simulink model "station_no_recovery"  (R2015a)
settings: Solver=ode45  StartTime=0  StopTime=5000  FixedStep=10  MaxStep=1  RelTol=1e-3
(part 2 of 4)

== system station_no_recovery/Восстанавливаемые объекты/ГТЭ-6//6,3/Subsystem1 ==
  λ1 : Inport
  λ2 : Inport  Port=2
  M : Inport  Port=3
  dP : Inport  Port=4
  Pz : Inport  Port=5
  dt : Inport  Port=6
  trec : Inport  Port=7
  t_start : Inport  Port=8
  Chart : Stateflow chart  TreatAsAtomicUnit=on
  Clock : Clock
  Data Store Memory : DataStoreMemory  DataStoreName=t4_1
  Data Store Read : DataStoreRead  DataStoreName=t4_1
  Data Store Write : DataStoreWrite  DataStoreName=t4_1
  Display : Display
  Element Exponential : Subsystem  mask(Element Exponential){}
      mask help:
      | <p>Возвращает вероятность безотказной работы невосстанавливаемого элемента
      | по экспоненциальному закону распределения.</p>
      | <p>Экспоненциальное (или показательное) распределение — абсолютно непрерывное
      | распределение, моделирующее время между двумя последовательными свершениями
      | одного и того же события.</p>
      | <p>Экспоненциальное распределение используют при оценке надежности сложных
      | технических систем, не подверженных износу и старению и в случаях, когда
      | отказы объектов имеют случайный характер.</p>
      mask Help:
      | <p>Возвращает вероятность безотказной работы невосстанавливаемого элемента по экспоненциальному
      | закону распределения.</p>
      | <p>Экспоненциальное распределение используют при оценке надежности сложных
      | технических систем, не подверженных износу и старению и в случаях, когда
      | отказы объектов имеют случайный характер.</p>
      | <p>Входной параметр λ - интенсивность событий в рассматриваемом потоке.</p>
      | <p>Выходной параметр P(t) - вероятность безотказной работы элемента.</p>
      mask Display:
      | image('images/png/exp.png')
      | port_label('input', 1, 'λ')
      | port_label('output', 1, 'P(t)')
  Element Normal : Subsystem  mask(Element Normal){}
      mask help:
      | <p>Возвращает вероятность безотказной работы невосстанавливаемого
      | элемента по нормальному закону распределения.</p>
      | <p>Нормальное распределение, также называемое распределением Гаусса или
      | Гаусса — Лапласа — распределение вероятностей, которое в одномерном
      | случае задаётся функцией плотности вероятности, совпадающей с функцией
      | Гаусса.</p>
      | <p>Нормальное распределение обычно используют при оценке надежности объектов,
      | основной причиной отказа которых является износ.</p>
      mask Help:
      | <p>Возвращает вероятность безотказной работы невосстанавливаемого
      | элемента по нормальному закону распределения.</p>
      | <p>Нормальное распределение обычно используют при оценке надежности объектов,
      | основной причиной отказа которых является износ.</p>
      | <p>Входные параметры:</p>
      | <p>λ - среднее квадратическое отклонение наработки до отказа,</p>
      | <p>М - математическое ожидание наработки до отказа.</p>
      | <p>Выходной параметр P(t) - вероятность безотказной работы элемента.</p>
      mask Display:
      | image('images/png/normal_nogrid.png')
      | port_label('input', 1, 'λ')
      | port_label('input', 2, 'M')
      | port_label('output', 1, 'P(t)')
  Сircuit Series : Subsystem  mask(Сircuit Series){}
      mask help:
      | <p>Возвращает вероятность безотказной работы двух последовательно соединенных
      | элементов.</p>
      | <p>В системе с последовательной структурой отказ любого компонента приводит
      | к отказу системы в целом.</p>
      mask Help:
      | <p>Возвращает вероятность безотказной работы двух последовательно соединенных
      | элементов.</p>
      | <p>Входные параметры:</p>
      | <p>P1 - вероятность безотказной работы первого элемента,</p>
      | <p>P2 - вероятность безотказной работы второго элемента.</p>
      | <p>Выходной параметр P12 - вероятность безотказной работы двух последовательно
      | соединенных элементов.</p>
      mask Display:
      | image('images/png/series2.png')
      | port_label('input', 1, 'P1')
      | port_label('input', 2, 'P2')
      | port_label('output', 1, 'P12')
  P : Outport
  wires:
  M/1 -> Element Normal/2("M ")
  dP/1 -> Chart/5(dP)
  Pz/1 -> Chart/3(Pz)
  λ1/1 -> Element Exponential/1("lambda ")
  dt/1 -> Chart/2(delta_t)
  Clock/1 -> Chart/6(t)
  λ2/1 -> Element Normal/1("lambda ")
  Chart/2(P) -> P/1
  Element Normal/1(P(t)) -> Сircuit Series/2(P2)
  Element Exponential/1(P(t)1) -> Сircuit Series/1(P1)
  Сircuit Series/1(P12) -> Chart/7(P0), Display/1
  trec/1 -> Chart/4(trec)
  Chart/1(tv) -> Data Store Write/1
  t_start/1 -> Chart/1(t_start)
  Data Store Read/1 -> Element Exponential/2(t), Element Normal/3(t)

== system station_no_recovery/Восстанавливаемые объекты/ГТЭ-6//6,3/Subsystem2 ==
  λ1 : Inport
  λ2 : Inport  Port=2
  M : Inport  Port=3
  dP : Inport  Port=4
  Pz : Inport  Port=5
  dt : Inport  Port=6
  trec : Inport  Port=7
  t_start : Inport  Port=8
  Chart : Stateflow chart  TreatAsAtomicUnit=on
  Clock : Clock
  Data Store Memory : DataStoreMemory  DataStoreName=t4_2
  Data Store Read : DataStoreRead  DataStoreName=t4_2
  Data Store Write : DataStoreWrite  DataStoreName=t4_2
  Display : Display
  Element Exponential : Subsystem  mask(Element Exponential){}
      mask help:
      | <p>Возвращает вероятность безотказной работы невосстанавливаемого элемента
      | по экспоненциальному закону распределения.</p>
      | <p>Экспоненциальное (или показательное) распределение — абсолютно непрерывное
      | распределение, моделирующее время между двумя последовательными свершениями
      | одного и того же события.</p>
      | <p>Экспоненциальное распределение используют при оценке надежности сложных
      | технических систем, не подверженных износу и старению и в случаях, когда
      | отказы объектов имеют случайный характер.</p>
      mask Help:
      | <p>Возвращает вероятность безотказной работы невосстанавливаемого элемента по экспоненциальному
      | закону распределения.</p>
      | <p>Экспоненциальное распределение используют при оценке надежности сложных
      | технических систем, не подверженных износу и старению и в случаях, когда
      | отказы объектов имеют случайный характер.</p>
      | <p>Входной параметр λ - интенсивность событий в рассматриваемом потоке.</p>
      | <p>Выходной параметр P(t) - вероятность безотказной работы элемента.</p>
      mask Display:
      | image('images/png/exp.png')
      | port_label('input', 1, 'λ')
      | port_label('output', 1, 'P(t)')
  Element Normal : Subsystem  mask(Element Normal){}
      mask help:
      | <p>Возвращает вероятность безотказной работы невосстанавливаемого
      | элемента по нормальному закону распределения.</p>
      | <p>Нормальное распределение, также называемое распределением Гаусса или
      | Гаусса — Лапласа — распределение вероятностей, которое в одномерном
      | случае задаётся функцией плотности вероятности, совпадающей с функцией
      | Гаусса.</p>
      | <p>Нормальное распределение обычно используют при оценке надежности объектов,
      | основной причиной отказа которых является износ.</p>
      mask Help:
      | <p>Возвращает вероятность безотказной работы невосстанавливаемого
      | элемента по нормальному закону распределения.</p>
      | <p>Нормальное распределение обычно используют при оценке надежности объектов,
      | основной причиной отказа которых является износ.</p>
      | <p>Входные параметры:</p>
      | <p>λ - среднее квадратическое отклонение наработки до отказа,</p>
      | <p>М - математическое ожидание наработки до отказа.</p>
      | <p>Выходной параметр P(t) - вероятность безотказной работы элемента.</p>
      mask Display:
      | image('images/png/normal_nogrid.png')
      | port_label('input', 1, 'λ')
      | port_label('input', 2, 'M')
      | port_label('output', 1, 'P(t)')
  Сircuit Series : Subsystem  mask(Сircuit Series){}
      mask help:
      | <p>Возвращает вероятность безотказной работы двух последовательно соединенных
      | элементов.</p>
      | <p>В системе с последовательной структурой отказ любого компонента приводит
      | к отказу системы в целом.</p>
      mask Help:
      | <p>Возвращает вероятность безотказной работы двух последовательно соединенных
      | элементов.</p>
      | <p>Входные параметры:</p>
      | <p>P1 - вероятность безотказной работы первого элемента,</p>
      | <p>P2 - вероятность безотказной работы второго элемента.</p>
      | <p>Выходной параметр P12 - вероятность безотказной работы двух последовательно
      | соединенных элементов.</p>
      mask Display:
      | image('images/png/series2.png')
      | port_label('input', 1, 'P1')
      | port_label('input', 2, 'P2')
      | port_label('output', 1, 'P12')
  P : Outport
  wires:
  Data Store Read/1 -> Element Normal/3(t), Element Exponential/2(t)
  t_start/1 -> Chart/1(t_start)
  Chart/1(tv) -> Data Store Write/1
  trec/1 -> Chart/4(trec)
  Сircuit Series/1(P12) -> Display/1, Chart/7(P0)
  Element Exponential/1(P(t)1) -> Сircuit Series/1(P1)
  Element Normal/1(P(t)) -> Сircuit Series/2(P2)
  Chart/2(P) -> P/1
  λ2/1 -> Element Normal/1("lambda ")
  Clock/1 -> Chart/6(t)
  dt/1 -> Chart/2(delta_t)
  λ1/1 -> Element Exponential/1("lambda ")
  Pz/1 -> Chart/3(Pz)
  dP/1 -> Chart/5(dP)
  M/1 -> Element Normal/2("M ")

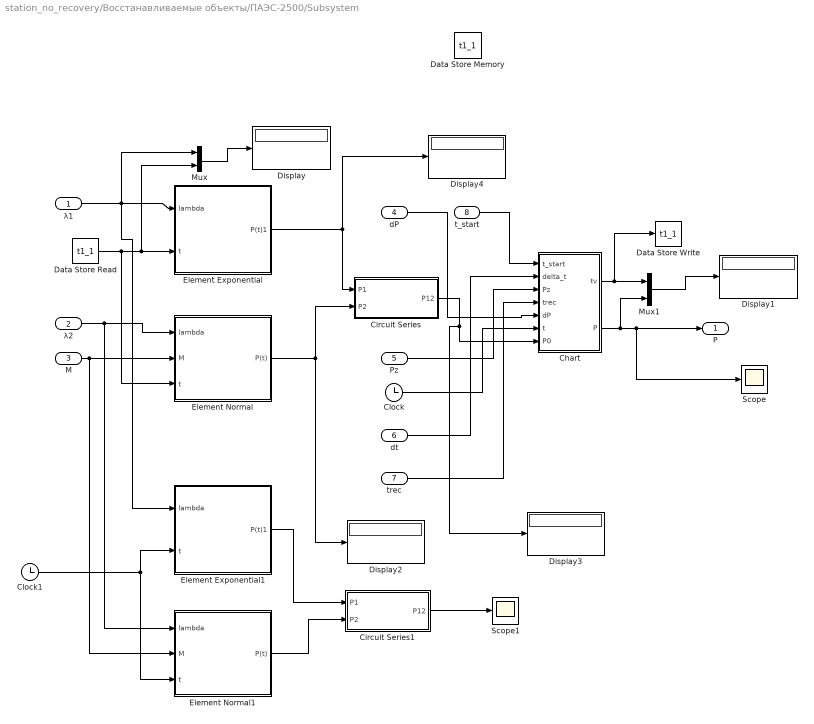
== system station_no_recovery/Восстанавливаемые объекты/ПАЭС-2500/Subsystem ==
  λ1 : Inport
  λ2 : Inport  Port=2
  M : Inport  Port=3
  dP : Inport  Port=4
  Pz : Inport  Port=5
  dt : Inport  Port=6
  trec : Inport  Port=7
  t_start : Inport  Port=8
  Chart : Stateflow chart  TreatAsAtomicUnit=on
  Clock : Clock
  Clock1 : Clock
  Data Store Memory : DataStoreMemory  DataStoreName=t1_1
  Data Store Read : DataStoreRead  DataStoreName=t1_1
  Data Store Write : DataStoreWrite  DataStoreName=t1_1
  Display{,1..4} (5 alike) : Display
  Element Exponential : Subsystem  mask(Element Exponential){}
      mask help:
      | <p>Возвращает вероятность безотказной работы невосстанавливаемого элемента
      | по экспоненциальному закону распределения.</p>
      | <p>Экспоненциальное (или показательное) распределение — абсолютно непрерывное
      | распределение, моделирующее время между двумя последовательными свершениями
      | одного и того же события.</p>
      | <p>Экспоненциальное распределение используют при оценке надежности сложных
      | технических систем, не подверженных износу и старению и в случаях, когда
      | отказы объектов имеют случайный характер.</p>
      mask Help:
      | <p>Возвращает вероятность безотказной работы невосстанавливаемого элемента по экспоненциальному
      | закону распределения.</p>
      | <p>Экспоненциальное распределение используют при оценке надежности сложных
      | технических систем, не подверженных износу и старению и в случаях, когда
      | отказы объектов имеют случайный характер.</p>
      | <p>Входной параметр λ - интенсивность событий в рассматриваемом потоке.</p>
      | <p>Выходной параметр P(t) - вероятность безотказной работы элемента.</p>
      mask Display:
      | image('images/png/exp.png')
      | port_label('input', 1, 'λ')
      | port_label('output', 1, 'P(t)')
  Element Exponential1 : Subsystem  mask(Element Exponential){}
      mask help:
      | <p>Возвращает вероятность безотказной работы невосстанавливаемого элемента
      | по экспоненциальному закону распределения.</p>
      | <p>Экспоненциальное (или показательное) распределение — абсолютно непрерывное
      | распределение, моделирующее время между двумя последовательными свершениями
      | одного и того же события.</p>
      | <p>Экспоненциальное распределение используют при оценке надежности сложных
      | технических систем, не подверженных износу и старению и в случаях, когда
      | отказы объектов имеют случайный характер.</p>
      mask Help:
      | <p>Возвращает вероятность безотказной работы невосстанавливаемого элемента по экспоненциальному
      | закону распределения.</p>
      | <p>Экспоненциальное распределение используют при оценке надежности сложных
      | технических систем, не подверженных износу и старению и в случаях, когда
      | отказы объектов имеют случайный характер.</p>
      | <p>Входной параметр λ - интенсивность событий в рассматриваемом потоке.</p>
      | <p>Выходной параметр P(t) - вероятность безотказной работы элемента.</p>
      mask Display:
      | image('images/png/exp.png')
      | port_label('input', 1, 'λ')
      | port_label('output', 1, 'P(t)')
  Element Normal : Subsystem  mask(Element Normal){}
      mask help:
      | <p>Возвращает вероятность безотказной работы невосстанавливаемого
      | элемента по нормальному закону распределения.</p>
      | <p>Нормальное распределение, также называемое распределением Гаусса или
      | Гаусса — Лапласа — распределение вероятностей, которое в одномерном
      | случае задаётся функцией плотности вероятности, совпадающей с функцией
      | Гаусса.</p>
      | <p>Нормальное распределение обычно используют при оценке надежности объектов,
      | основной причиной отказа которых является износ.</p>
      mask Help:
      | <p>Возвращает вероятность безотказной работы невосстанавливаемого
      | элемента по нормальному закону распределения.</p>
      | <p>Нормальное распределение обычно используют при оценке надежности объектов,
      | основной причиной отказа которых является износ.</p>
      | <p>Входные параметры:</p>
      | <p>λ - среднее квадратическое отклонение наработки до отказа,</p>
      | <p>М - математическое ожидание наработки до отказа.</p>
      | <p>Выходной параметр P(t) - вероятность безотказной работы элемента.</p>
      mask Display:
      | image('images/png/normal_nogrid.png')
      | port_label('input', 1, 'λ')
      | port_label('input', 2, 'M')
      | port_label('output', 1, 'P(t)')
  Element Normal1 : Subsystem  mask(Element Normal){}
      mask help:
      | <p>Возвращает вероятность безотказной работы невосстанавливаемого
      | элемента по нормальному закону распределения.</p>
      | <p>Нормальное распределение, также называемое распределением Гаусса или
      | Гаусса — Лапласа — распределение вероятностей, которое в одномерном
      | случае задаётся функцией плотности вероятности, совпадающей с функцией
      | Гаусса.</p>
      | <p>Нормальное распределение обычно используют при оценке надежности объектов,
      | основной причиной отказа которых является износ.</p>
      mask Help:
      | <p>Возвращает вероятность безотказной работы невосстанавливаемого
      | элемента по нормальному закону распределения.</p>
      | <p>Нормальное распределение обычно используют при оценке надежности объектов,
      | основной причиной отказа которых является износ.</p>
      | <p>Входные параметры:</p>
      | <p>λ - среднее квадратическое отклонение наработки до отказа,</p>
      | <p>М - математическое ожидание наработки до отказа.</p>
      | <p>Выходной параметр P(t) - вероятность безотказной работы элемента.</p>
      mask Display:
      | image('images/png/normal_nogrid.png')
      | port_label('input', 1, 'λ')
      | port_label('input', 2, 'M')
      | port_label('output', 1, 'P(t)')
  Mux : Mux  Inputs=2
  Mux1 : Mux  Inputs=2
  Scope : Scope
  Scope1 : Scope
      settings: SaveName=ScopeData2
  Сircuit Series : Subsystem  mask(Сircuit Series){}
      mask help:
      | <p>Возвращает вероятность безотказной работы двух последовательно соединенных
      | элементов.</p>
      | <p>В системе с последовательной структурой отказ любого компонента приводит
      | к отказу системы в целом.</p>
      mask Help:
      | <p>Возвращает вероятность безотказной работы двух последовательно соединенных
      | элементов.</p>
      | <p>Входные параметры:</p>
      | <p>P1 - вероятность безотказной работы первого элемента,</p>
      | <p>P2 - вероятность безотказной работы второго элемента.</p>
      | <p>Выходной параметр P12 - вероятность безотказной работы двух последовательно
      | соединенных элементов.</p>
      mask Display:
      | image('images/png/series2.png')
      | port_label('input', 1, 'P1')
      | port_label('input', 2, 'P2')
      | port_label('output', 1, 'P12')
  Сircuit Series1 : Subsystem  mask(Сircuit Series){}
      mask help:
      | <p>Возвращает вероятность безотказной работы двух последовательно соединенных
      | элементов.</p>
      | <p>В системе с последовательной структурой отказ любого компонента приводит
      | к отказу системы в целом.</p>
      mask Help:
      | <p>Возвращает вероятность безотказной работы двух последовательно соединенных
      | элементов.</p>
      | <p>Входные параметры:</p>
      | <p>P1 - вероятность безотказной работы первого элемента,</p>
      | <p>P2 - вероятность безотказной работы второго элемента.</p>
      | <p>Выходной параметр P12 - вероятность безотказной работы двух последовательно
      | соединенных элементов.</p>
      mask Display:
      | image('images/png/series2.png')
      | port_label('input', 1, 'P1')
      | port_label('input', 2, 'P2')
      | port_label('output', 1, 'P12')
  P : Outport
  wires:
  Element Exponential/1(P(t)1) -> Сircuit Series/1(P1), Display4/1
  Element Normal/1(P(t)) -> Сircuit Series/2(P2), Display2/1
  Chart/1(tv) -> Data Store Write/1, Mux1/1
  Chart/2(P) -> Mux1/2, Scope/1, P/1
  λ2/1 -> Element Normal1/1("lambda "), Element Normal/1("lambda ")
  Сircuit Series/1(P12) -> Chart/7(P0), Display3/1
  λ1/1 -> Element Exponential1/1("lambda "), Mux/1, Element Exponential/1("lambda ")
  M/1 -> Element Normal1/2("M "), Element Normal/2("M ")
  Mux/1 -> Display/1
  Mux1/1 -> Display1/1
  t_start/1 -> Chart/1(t_start)
  dt/1 -> Chart/2(delta_t)
  Pz/1 -> Chart/3(Pz)
  trec/1 -> Chart/4(trec)
  Clock/1 -> Chart/6(t)
  dP/1 -> Chart/5(dP)
  Data Store Read/1 -> Element Normal/3(t), Mux/2, Element Exponential/2(t)
  Clock1/1 -> Element Normal1/3(t), Element Exponential1/2(t)
  Element Exponential1/1(P(t)1) -> Сircuit Series1/1(P1)
  Element Normal1/1(P(t)) -> Сircuit Series1/2(P2)
  Сircuit Series1/1(P12) -> Scope1/1

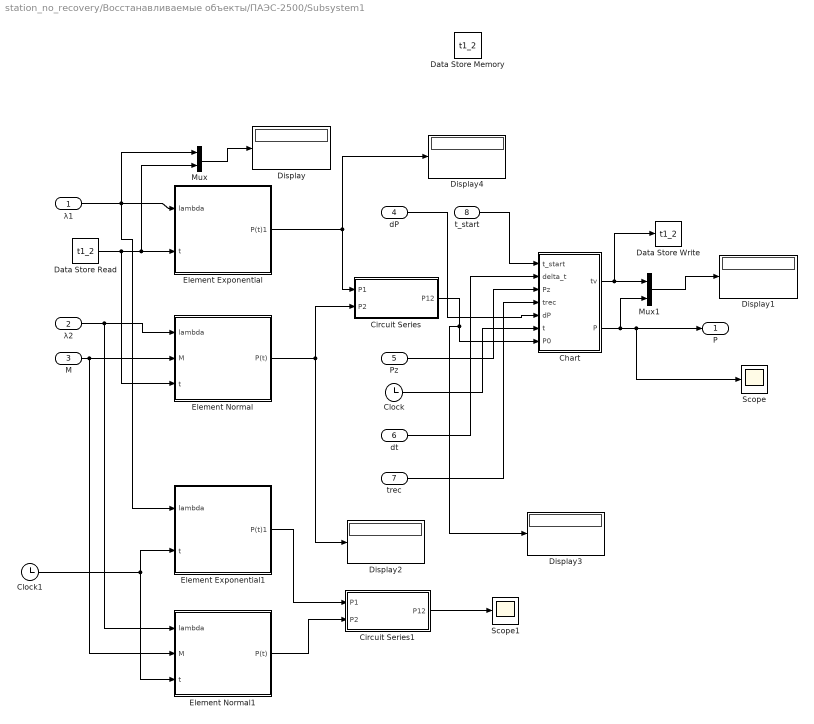
== system station_no_recovery/Восстанавливаемые объекты/ПАЭС-2500/Subsystem1 ==
  λ1 : Inport
  λ2 : Inport  Port=2
  M : Inport  Port=3
  dP : Inport  Port=4
  Pz : Inport  Port=5
  dt : Inport  Port=6
  trec : Inport  Port=7
  t_start : Inport  Port=8
  Chart : Stateflow chart  TreatAsAtomicUnit=on
  Clock : Clock
  Clock1 : Clock
  Data Store Memory : DataStoreMemory  DataStoreName=t1_2
  Data Store Read : DataStoreRead  DataStoreName=t1_2
  Data Store Write : DataStoreWrite  DataStoreName=t1_2
  Display{,1..4} (5 alike) : Display
  Element Exponential : Subsystem  mask(Element Exponential){}
      mask help:
      | <p>Возвращает вероятность безотказной работы невосстанавливаемого элемента
      | по экспоненциальному закону распределения.</p>
      | <p>Экспоненциальное (или показательное) распределение — абсолютно непрерывное
      | распределение, моделирующее время между двумя последовательными свершениями
      | одного и того же события.</p>
      | <p>Экспоненциальное распределение используют при оценке надежности сложных
      | технических систем, не подверженных износу и старению и в случаях, когда
      | отказы объектов имеют случайный характер.</p>
      mask Help:
      | <p>Возвращает вероятность безотказной работы невосстанавливаемого элемента по экспоненциальному
      | закону распределения.</p>
      | <p>Экспоненциальное распределение используют при оценке надежности сложных
      | технических систем, не подверженных износу и старению и в случаях, когда
      | отказы объектов имеют случайный характер.</p>
      | <p>Входной параметр λ - интенсивность событий в рассматриваемом потоке.</p>
      | <p>Выходной параметр P(t) - вероятность безотказной работы элемента.</p>
      mask Display:
      | image('images/png/exp.png')
      | port_label('input', 1, 'λ')
      | port_label('output', 1, 'P(t)')
  Element Exponential1 : Subsystem  mask(Element Exponential){}
      mask help:
      | <p>Возвращает вероятность безотказной работы невосстанавливаемого элемента
      | по экспоненциальному закону распределения.</p>
      | <p>Экспоненциальное (или показательное) распределение — абсолютно непрерывное
      | распределение, моделирующее время между двумя последовательными свершениями
      | одного и того же события.</p>
      | <p>Экспоненциальное распределение используют при оценке надежности сложных
      | технических систем, не подверженных износу и старению и в случаях, когда
      | отказы объектов имеют случайный характер.</p>
      mask Help:
      | <p>Возвращает вероятность безотказной работы невосстанавливаемого элемента по экспоненциальному
      | закону распределения.</p>
      | <p>Экспоненциальное распределение используют при оценке надежности сложных
      | технических систем, не подверженных износу и старению и в случаях, когда
      | отказы объектов имеют случайный характер.</p>
      | <p>Входной параметр λ - интенсивность событий в рассматриваемом потоке.</p>
      | <p>Выходной параметр P(t) - вероятность безотказной работы элемента.</p>
      mask Display:
      | image('images/png/exp.png')
      | port_label('input', 1, 'λ')
      | port_label('output', 1, 'P(t)')
  Element Normal : Subsystem  mask(Element Normal){}
      mask help:
      | <p>Возвращает вероятность безотказной работы невосстанавливаемого
      | элемента по нормальному закону распределения.</p>
      | <p>Нормальное распределение, также называемое распределением Гаусса или
      | Гаусса — Лапласа — распределение вероятностей, которое в одномерном
      | случае задаётся функцией плотности вероятности, совпадающей с функцией
      | Гаусса.</p>
      | <p>Нормальное распределение обычно используют при оценке надежности объектов,
      | основной причиной отказа которых является износ.</p>
      mask Help:
      | <p>Возвращает вероятность безотказной работы невосстанавливаемого
      | элемента по нормальному закону распределения.</p>
      | <p>Нормальное распределение обычно используют при оценке надежности объектов,
      | основной причиной отказа которых является износ.</p>
      | <p>Входные параметры:</p>
      | <p>λ - среднее квадратическое отклонение наработки до отказа,</p>
      | <p>М - математическое ожидание наработки до отказа.</p>
      | <p>Выходной параметр P(t) - вероятность безотказной работы элемента.</p>
      mask Display:
      | image('images/png/normal_nogrid.png')
      | port_label('input', 1, 'λ')
      | port_label('input', 2, 'M')
      | port_label('output', 1, 'P(t)')
  Element Normal1 : Subsystem  mask(Element Normal){}
      mask help:
      | <p>Возвращает вероятность безотказной работы невосстанавливаемого
      | элемента по нормальному закону распределения.</p>
      | <p>Нормальное распределение, также называемое распределением Гаусса или
      | Гаусса — Лапласа — распределение вероятностей, которое в одномерном
      | случае задаётся функцией плотности вероятности, совпадающей с функцией
      | Гаусса.</p>
      | <p>Нормальное распределение обычно используют при оценке надежности объектов,
      | основной причиной отказа которых является износ.</p>
      mask Help:
      | <p>Возвращает вероятность безотказной работы невосстанавливаемого
      | элемента по нормальному закону распределения.</p>
      | <p>Нормальное распределение обычно используют при оценке надежности объектов,
      | основной причиной отказа которых является износ.</p>
      | <p>Входные параметры:</p>
      | <p>λ - среднее квадратическое отклонение наработки до отказа,</p>
      | <p>М - математическое ожидание наработки до отказа.</p>
      | <p>Выходной параметр P(t) - вероятность безотказной работы элемента.</p>
      mask Display:
      | image('images/png/normal_nogrid.png')
      | port_label('input', 1, 'λ')
      | port_label('input', 2, 'M')
      | port_label('output', 1, 'P(t)')
  Mux : Mux  Inputs=2
  Mux1 : Mux  Inputs=2
  Scope : Scope
  Scope1 : Scope
      settings: SaveName=ScopeData2
  Сircuit Series : Subsystem  mask(Сircuit Series){}
      mask help:
      | <p>Возвращает вероятность безотказной работы двух последовательно соединенных
      | элементов.</p>
      | <p>В системе с последовательной структурой отказ любого компонента приводит
      | к отказу системы в целом.</p>
      mask Help:
      | <p>Возвращает вероятность безотказной работы двух последовательно соединенных
      | элементов.</p>
      | <p>Входные параметры:</p>
      | <p>P1 - вероятность безотказной работы первого элемента,</p>
      | <p>P2 - вероятность безотказной работы второго элемента.</p>
      | <p>Выходной параметр P12 - вероятность безотказной работы двух последовательно
      | соединенных элементов.</p>
      mask Display:
      | image('images/png/series2.png')
      | port_label('input', 1, 'P1')
      | port_label('input', 2, 'P2')
      | port_label('output', 1, 'P12')
  Сircuit Series1 : Subsystem  mask(Сircuit Series){}
      mask help:
      | <p>Возвращает вероятность безотказной работы двух последовательно соединенных
      | элементов.</p>
      | <p>В системе с последовательной структурой отказ любого компонента приводит
      | к отказу системы в целом.</p>
      mask Help:
      | <p>Возвращает вероятность безотказной работы двух последовательно соединенных
      | элементов.</p>
      | <p>Входные параметры:</p>
      | <p>P1 - вероятность безотказной работы первого элемента,</p>
      | <p>P2 - вероятность безотказной работы второго элемента.</p>
      | <p>Выходной параметр P12 - вероятность безотказной работы двух последовательно
      | соединенных элементов.</p>
      mask Display:
      | image('images/png/series2.png')
      | port_label('input', 1, 'P1')
      | port_label('input', 2, 'P2')
      | port_label('output', 1, 'P12')
  P : Outport
  wires:
  Сircuit Series1/1(P12) -> Scope1/1
  Element Normal1/1(P(t)) -> Сircuit Series1/2(P2)
  Element Exponential1/1(P(t)1) -> Сircuit Series1/1(P1)
  Clock1/1 -> Element Exponential1/2(t), Element Normal1/3(t)
  Data Store Read/1 -> Element Exponential/2(t), Mux/2, Element Normal/3(t)
  dP/1 -> Chart/5(dP)
  Clock/1 -> Chart/6(t)
  trec/1 -> Chart/4(trec)
  Pz/1 -> Chart/3(Pz)
  dt/1 -> Chart/2(delta_t)
  t_start/1 -> Chart/1(t_start)
  Mux1/1 -> Display1/1
  Mux/1 -> Display/1
  M/1 -> Element Normal/2("M "), Element Normal1/2("M ")
  λ1/1 -> Element Exponential/1("lambda "), Mux/1, Element Exponential1/1("lambda ")
  Сircuit Series/1(P12) -> Display3/1, Chart/7(P0)
  λ2/1 -> Element Normal/1("lambda "), Element Normal1/1("lambda ")
  Chart/2(P) -> P/1, Scope/1, Mux1/2
  Chart/1(tv) -> Mux1/1, Data Store Write/1
  Element Normal/1(P(t)) -> Display2/1, Сircuit Series/2(P2)
  Element Exponential/1(P(t)1) -> Display4/1, Сircuit Series/1(P1)

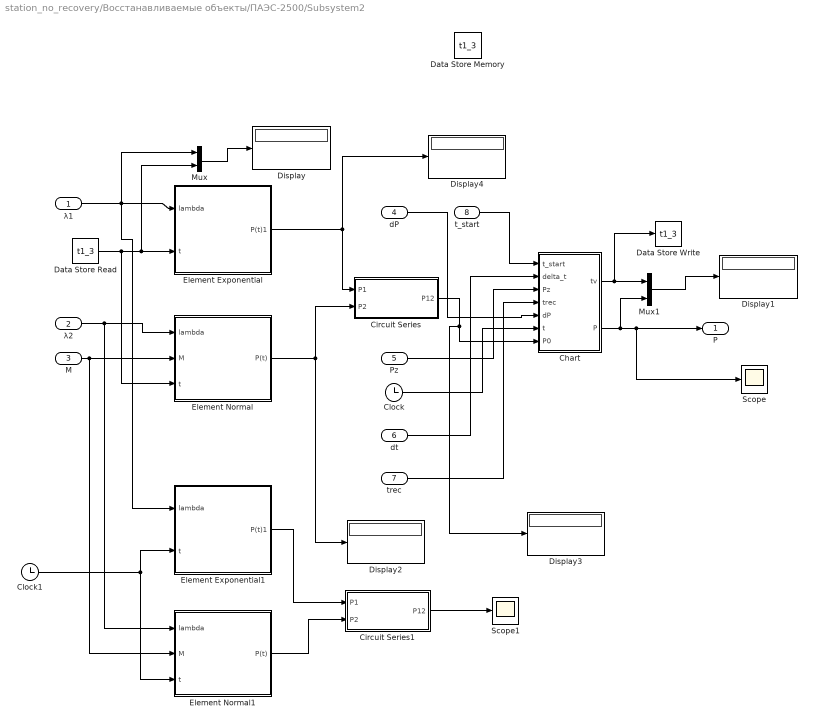
== system station_no_recovery/Восстанавливаемые объекты/ПАЭС-2500/Subsystem2 ==
  λ1 : Inport
  λ2 : Inport  Port=2
  M : Inport  Port=3
  dP : Inport  Port=4
  Pz : Inport  Port=5
  dt : Inport  Port=6
  trec : Inport  Port=7
  t_start : Inport  Port=8
  Chart : Stateflow chart  TreatAsAtomicUnit=on
  Clock : Clock
  Clock1 : Clock
  Data Store Memory : DataStoreMemory  DataStoreName=t1_3
  Data Store Read : DataStoreRead  DataStoreName=t1_3
  Data Store Write : DataStoreWrite  DataStoreName=t1_3
  Display{,1..4} (5 alike) : Display
  Element Exponential : Subsystem  mask(Element Exponential){}
      mask help:
      | <p>Возвращает вероятность безотказной работы невосстанавливаемого элемента
      | по экспоненциальному закону распределения.</p>
      | <p>Экспоненциальное (или показательное) распределение — абсолютно непрерывное
      | распределение, моделирующее время между двумя последовательными свершениями
      | одного и того же события.</p>
      | <p>Экспоненциальное распределение используют при оценке надежности сложных
      | технических систем, не подверженных износу и старению и в случаях, когда
      | отказы объектов имеют случайный характер.</p>
      mask Help:
      | <p>Возвращает вероятность безотказной работы невосстанавливаемого элемента по экспоненциальному
      | закону распределения.</p>
      | <p>Экспоненциальное распределение используют при оценке надежности сложных
      | технических систем, не подверженных износу и старению и в случаях, когда
      | отказы объектов имеют случайный характер.</p>
      | <p>Входной параметр λ - интенсивность событий в рассматриваемом потоке.</p>
      | <p>Выходной параметр P(t) - вероятность безотказной работы элемента.</p>
      mask Display:
      | image('images/png/exp.png')
      | port_label('input', 1, 'λ')
      | port_label('output', 1, 'P(t)')
  Element Exponential1 : Subsystem  mask(Element Exponential){}
      mask help:
      | <p>Возвращает вероятность безотказной работы невосстанавливаемого элемента
      | по экспоненциальному закону распределения.</p>
      | <p>Экспоненциальное (или показательное) распределение — абсолютно непрерывное
      | распределение, моделирующее время между двумя последовательными свершениями
      | одного и того же события.</p>
      | <p>Экспоненциальное распределение используют при оценке надежности сложных
      | технических систем, не подверженных износу и старению и в случаях, когда
      | отказы объектов имеют случайный характер.</p>
      mask Help:
      | <p>Возвращает вероятность безотказной работы невосстанавливаемого элемента по экспоненциальному
      | закону распределения.</p>
      | <p>Экспоненциальное распределение используют при оценке надежности сложных
      | технических систем, не подверженных износу и старению и в случаях, когда
      | отказы объектов имеют случайный характер.</p>
      | <p>Входной параметр λ - интенсивность событий в рассматриваемом потоке.</p>
      | <p>Выходной параметр P(t) - вероятность безотказной работы элемента.</p>
      mask Display:
      | image('images/png/exp.png')
      | port_label('input', 1, 'λ')
      | port_label('output', 1, 'P(t)')
  Element Normal : Subsystem  mask(Element Normal){}
      mask help:
      | <p>Возвращает вероятность безотказной работы невосстанавливаемого
      | элемента по нормальному закону распределения.</p>
      | <p>Нормальное распределение, также называемое распределением Гаусса или
      | Гаусса — Лапласа — распределение вероятностей, которое в одномерном
      | случае задаётся функцией плотности вероятности, совпадающей с функцией
      | Гаусса.</p>
      | <p>Нормальное распределение обычно используют при оценке надежности объектов,
      | основной причиной отказа которых является износ.</p>
      mask Help:
      | <p>Возвращает вероятность безотказной работы невосстанавливаемого
      | элемента по нормальному закону распределения.</p>
      | <p>Нормальное распределение обычно используют при оценке надежности объектов,
      | основной причиной отказа которых является износ.</p>
      | <p>Входные параметры:</p>
      | <p>λ - среднее квадратическое отклонение наработки до отказа,</p>
      | <p>М - математическое ожидание наработки до отказа.</p>
      | <p>Выходной параметр P(t) - вероятность безотказной работы элемента.</p>
      mask Display:
      | image('images/png/normal_nogrid.png')
      | port_label('input', 1, 'λ')
      | port_label('input', 2, 'M')
      | port_label('output', 1, 'P(t)')
  Element Normal1 : Subsystem  mask(Element Normal){}
      mask help:
      | <p>Возвращает вероятность безотказной работы невосстанавливаемого
      | элемента по нормальному закону распределения.</p>
      | <p>Нормальное распределение, также называемое распределением Гаусса или
      | Гаусса — Лапласа — распределение вероятностей, которое в одномерном
      | случае задаётся функцией плотности вероятности, совпадающей с функцией
      | Гаусса.</p>
      | <p>Нормальное распределение обычно используют при оценке надежности объектов,
      | основной причиной отказа которых является износ.</p>
      mask Help:
      | <p>Возвращает вероятность безотказной работы невосстанавливаемого
      | элемента по нормальному закону распределения.</p>
      | <p>Нормальное распределение обычно используют при оценке надежности объектов,
      | основной причиной отказа которых является износ.</p>
      | <p>Входные параметры:</p>
      | <p>λ - среднее квадратическое отклонение наработки до отказа,</p>
      | <p>М - математическое ожидание наработки до отказа.</p>
      | <p>Выходной параметр P(t) - вероятность безотказной работы элемента.</p>
      mask Display:
      | image('images/png/normal_nogrid.png')
      | port_label('input', 1, 'λ')
      | port_label('input', 2, 'M')
      | port_label('output', 1, 'P(t)')
  Mux : Mux  Inputs=2
  Mux1 : Mux  Inputs=2
  Scope : Scope
  Scope1 : Scope
      settings: SaveName=ScopeData2
  Сircuit Series : Subsystem  mask(Сircuit Series){}
      mask help:
      | <p>Возвращает вероятность безотказной работы двух последовательно соединенных
      | элементов.</p>
      | <p>В системе с последовательной структурой отказ любого компонента приводит
      | к отказу системы в целом.</p>
      mask Help:
      | <p>Возвращает вероятность безотказной работы двух последовательно соединенных
      | элементов.</p>
      | <p>Входные параметры:</p>
      | <p>P1 - вероятность безотказной работы первого элемента,</p>
      | <p>P2 - вероятность безотказной работы второго элемента.</p>
      | <p>Выходной параметр P12 - вероятность безотказной работы двух последовательно
      | соединенных элементов.</p>
      mask Display:
      | image('images/png/series2.png')
      | port_label('input', 1, 'P1')
      | port_label('input', 2, 'P2')
      | port_label('output', 1, 'P12')
  Сircuit Series1 : Subsystem  mask(Сircuit Series){}
      mask help:
      | <p>Возвращает вероятность безотказной работы двух последовательно соединенных
      | элементов.</p>
      | <p>В системе с последовательной структурой отказ любого компонента приводит
      | к отказу системы в целом.</p>
      mask Help:
      | <p>Возвращает вероятность безотказной работы двух последовательно соединенных
      | элементов.</p>
      | <p>Входные параметры:</p>
      | <p>P1 - вероятность безотказной работы первого элемента,</p>
      | <p>P2 - вероятность безотказной работы второго элемента.</p>
      | <p>Выходной параметр P12 - вероятность безотказной работы двух последовательно
      | соединенных элементов.</p>
      mask Display:
      | image('images/png/series2.png')
      | port_label('input', 1, 'P1')
      | port_label('input', 2, 'P2')
      | port_label('output', 1, 'P12')
  P : Outport
  wires:
  Сircuit Series1/1(P12) -> Scope1/1
  Element Normal1/1(P(t)) -> Сircuit Series1/2(P2)
  Element Exponential1/1(P(t)1) -> Сircuit Series1/1(P1)
  Clock1/1 -> Element Exponential1/2(t), Element Normal1/3(t)
  Data Store Read/1 -> Element Exponential/2(t), Mux/2, Element Normal/3(t)
  dP/1 -> Chart/5(dP)
  Clock/1 -> Chart/6(t)
  trec/1 -> Chart/4(trec)
  Pz/1 -> Chart/3(Pz)
  dt/1 -> Chart/2(delta_t)
  t_start/1 -> Chart/1(t_start)
  Mux1/1 -> Display1/1
  Mux/1 -> Display/1
  M/1 -> Element Normal/2("M "), Element Normal1/2("M ")
  λ1/1 -> Element Exponential/1("lambda "), Mux/1, Element Exponential1/1("lambda ")
  Сircuit Series/1(P12) -> Display3/1, Chart/7(P0)
  λ2/1 -> Element Normal/1("lambda "), Element Normal1/1("lambda ")
  Chart/2(P) -> P/1, Scope/1, Mux1/2
  Chart/1(tv) -> Mux1/1, Data Store Write/1
  Element Normal/1(P(t)) -> Display2/1, Сircuit Series/2(P2)
  Element Exponential/1(P(t)1) -> Display4/1, Сircuit Series/1(P1)

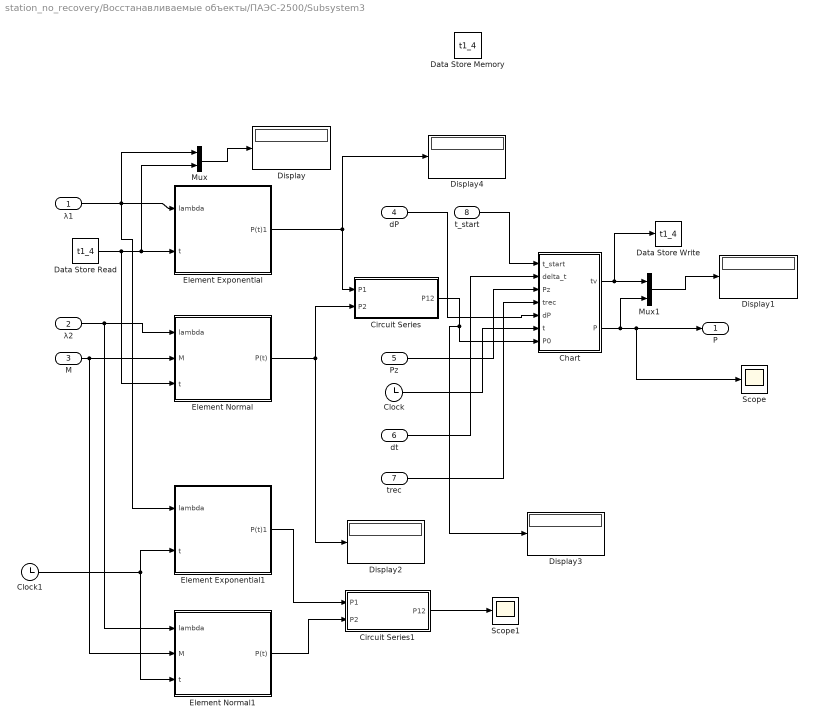
== system station_no_recovery/Восстанавливаемые объекты/ПАЭС-2500/Subsystem3 ==
  λ1 : Inport
  λ2 : Inport  Port=2
  M : Inport  Port=3
  dP : Inport  Port=4
  Pz : Inport  Port=5
  dt : Inport  Port=6
  trec : Inport  Port=7
  t_start : Inport  Port=8
  Chart : Stateflow chart  TreatAsAtomicUnit=on
  Clock : Clock
  Clock1 : Clock
  Data Store Memory : DataStoreMemory  DataStoreName=t1_4
  Data Store Read : DataStoreRead  DataStoreName=t1_4
  Data Store Write : DataStoreWrite  DataStoreName=t1_4
  Display{,1..4} (5 alike) : Display
  Element Exponential : Subsystem  mask(Element Exponential){}
      mask help:
      | <p>Возвращает вероятность безотказной работы невосстанавливаемого элемента
      | по экспоненциальному закону распределения.</p>
      | <p>Экспоненциальное (или показательное) распределение — абсолютно непрерывное
      | распределение, моделирующее время между двумя последовательными свершениями
      | одного и того же события.</p>
      | <p>Экспоненциальное распределение используют при оценке надежности сложных
      | технических систем, не подверженных износу и старению и в случаях, когда
      | отказы объектов имеют случайный характер.</p>
      mask Help:
      | <p>Возвращает вероятность безотказной работы невосстанавливаемого элемента по экспоненциальному
      | закону распределения.</p>
      | <p>Экспоненциальное распределение используют при оценке надежности сложных
      | технических систем, не подверженных износу и старению и в случаях, когда
      | отказы объектов имеют случайный характер.</p>
      | <p>Входной параметр λ - интенсивность событий в рассматриваемом потоке.</p>
      | <p>Выходной параметр P(t) - вероятность безотказной работы элемента.</p>
      mask Display:
      | image('images/png/exp.png')
      | port_label('input', 1, 'λ')
      | port_label('output', 1, 'P(t)')
  Element Exponential1 : Subsystem  mask(Element Exponential){}
      mask help:
      | <p>Возвращает вероятность безотказной работы невосстанавливаемого элемента
      | по экспоненциальному закону распределения.</p>
      | <p>Экспоненциальное (или показательное) распределение — абсолютно непрерывное
      | распределение, моделирующее время между двумя последовательными свершениями
      | одного и того же события.</p>
      | <p>Экспоненциальное распределение используют при оценке надежности сложных
      | технических систем, не подверженных износу и старению и в случаях, когда
      | отказы объектов имеют случайный характер.</p>
      mask Help:
      | <p>Возвращает вероятность безотказной работы невосстанавливаемого элемента по экспоненциальному
      | закону распределения.</p>
      | <p>Экспоненциальное распределение используют при оценке надежности сложных
      | технических систем, не подверженных износу и старению и в случаях, когда
      | отказы объектов имеют случайный характер.</p>
      | <p>Входной параметр λ - интенсивность событий в рассматриваемом потоке.</p>
      | <p>Выходной параметр P(t) - вероятность безотказной работы элемента.</p>
      mask Display:
      | image('images/png/exp.png')
      | port_label('input', 1, 'λ')
      | port_label('output', 1, 'P(t)')
  Element Normal : Subsystem  mask(Element Normal){}
      mask help:
      | <p>Возвращает вероятность безотказной работы невосстанавливаемого
      | элемента по нормальному закону распределения.</p>
      | <p>Нормальное распределение, также называемое распределением Гаусса или
      | Гаусса — Лапласа — распределение вероятностей, которое в одномерном
      | случае задаётся функцией плотности вероятности, совпадающей с функцией
      | Гаусса.</p>
      | <p>Нормальное распределение обычно используют при оценке надежности объектов,
      | основной причиной отказа которых является износ.</p>
      mask Help:
      | <p>Возвращает вероятность безотказной работы невосстанавливаемого
      | элемента по нормальному закону распределения.</p>
      | <p>Нормальное распределение обычно используют при оценке надежности объектов,
      | основной причиной отказа которых является износ.</p>
      | <p>Входные параметры:</p>
      | <p>λ - среднее квадратическое отклонение наработки до отказа,</p>
      | <p>М - математическое ожидание наработки до отказа.</p>
      | <p>Выходной параметр P(t) - вероятность безотказной работы элемента.</p>
      mask Display:
      | image('images/png/normal_nogrid.png')
      | port_label('input', 1, 'λ')
      | port_label('input', 2, 'M')
      | port_label('output', 1, 'P(t)')
  Element Normal1 : Subsystem  mask(Element Normal){}
      mask help:
      | <p>Возвращает вероятность безотказной работы невосстанавливаемого
      | элемента по нормальному закону распределения.</p>
      | <p>Нормальное распределение, также называемое распределением Гаусса или
      | Гаусса — Лапласа — распределение вероятностей, которое в одномерном
      | случае задаётся функцией плотности вероятности, совпадающей с функцией
      | Гаусса.</p>
      | <p>Нормальное распределение обычно используют при оценке надежности объектов,
      | основной причиной отказа которых является износ.</p>
      mask Help:
      | <p>Возвращает вероятность безотказной работы невосстанавливаемого
      | элемента по нормальному закону распределения.</p>
      | <p>Нормальное распределение обычно используют при оценке надежности объектов,
      | основной причиной отказа которых является износ.</p>
      | <p>Входные параметры:</p>
      | <p>λ - среднее квадратическое отклонение наработки до отказа,</p>
      | <p>М - математическое ожидание наработки до отказа.</p>
      | <p>Выходной параметр P(t) - вероятность безотказной работы элемента.</p>
      mask Display:
      | image('images/png/normal_nogrid.png')
      | port_label('input', 1, 'λ')
      | port_label('input', 2, 'M')
      | port_label('output', 1, 'P(t)')
  Mux : Mux  Inputs=2
  Mux1 : Mux  Inputs=2
  Scope : Scope
  Scope1 : Scope
      settings: SaveName=ScopeData2
  Сircuit Series : Subsystem  mask(Сircuit Series){}
      mask help:
      | <p>Возвращает вероятность безотказной работы двух последовательно соединенных
      | элементов.</p>
      | <p>В системе с последовательной структурой отказ любого компонента приводит
      | к отказу системы в целом.</p>
      mask Help:
      | <p>Возвращает вероятность безотказной работы двух последовательно соединенных
      | элементов.</p>
      | <p>Входные параметры:</p>
      | <p>P1 - вероятность безотказной работы первого элемента,</p>
      | <p>P2 - вероятность безотказной работы второго элемента.</p>
      | <p>Выходной параметр P12 - вероятность безотказной работы двух последовательно
      | соединенных элементов.</p>
      mask Display:
      | image('images/png/series2.png')
      | port_label('input', 1, 'P1')
      | port_label('input', 2, 'P2')
      | port_label('output', 1, 'P12')
  Сircuit Series1 : Subsystem  mask(Сircuit Series){}
      mask help:
      | <p>Возвращает вероятность безотказной работы двух последовательно соединенных
      | элементов.</p>
      | <p>В системе с последовательной структурой отказ любого компонента приводит
      | к отказу системы в целом.</p>
      mask Help:
      | <p>Возвращает вероятность безотказной работы двух последовательно соединенных
      | элементов.</p>
      | <p>Входные параметры:</p>
      | <p>P1 - вероятность безотказной работы первого элемента,</p>
      | <p>P2 - вероятность безотказной работы второго элемента.</p>
      | <p>Выходной параметр P12 - вероятность безотказной работы двух последовательно
      | соединенных элементов.</p>
      mask Display:
      | image('images/png/series2.png')
      | port_label('input', 1, 'P1')
      | port_label('input', 2, 'P2')
      | port_label('output', 1, 'P12')
  P : Outport
  wires:
  Element Exponential/1(P(t)1) -> Сircuit Series/1(P1), Display4/1
  Element Normal/1(P(t)) -> Сircuit Series/2(P2), Display2/1
  Chart/1(tv) -> Data Store Write/1, Mux1/1
  Chart/2(P) -> Mux1/2, Scope/1, P/1
  λ2/1 -> Element Normal1/1("lambda "), Element Normal/1("lambda ")
  Сircuit Series/1(P12) -> Chart/7(P0), Display3/1
  λ1/1 -> Element Exponential1/1("lambda "), Mux/1, Element Exponential/1("lambda ")
  M/1 -> Element Normal1/2("M "), Element Normal/2("M ")
  Mux/1 -> Display/1
  Mux1/1 -> Display1/1
  t_start/1 -> Chart/1(t_start)
  dt/1 -> Chart/2(delta_t)
  Pz/1 -> Chart/3(Pz)
  trec/1 -> Chart/4(trec)
  Clock/1 -> Chart/6(t)
  dP/1 -> Chart/5(dP)
  Data Store Read/1 -> Element Normal/3(t), Mux/2, Element Exponential/2(t)
  Clock1/1 -> Element Normal1/3(t), Element Exponential1/2(t)
  Element Exponential1/1(P(t)1) -> Сircuit Series1/1(P1)
  Element Normal1/1(P(t)) -> Сircuit Series1/2(P2)
  Сircuit Series1/1(P12) -> Scope1/1

== system station_no_recovery/Восстанавливаемые объекты/САТУРН/Subsystem1 ==
  λ1 : Inport
  λ2 : Inport  Port=2
  M : Inport  Port=3
  dP : Inport  Port=4
  Pz : Inport  Port=5
  dt : Inport  Port=6
  trec : Inport  Port=7
  t_start : Inport  Port=8
  Chart : Stateflow chart  TreatAsAtomicUnit=on
  Clock : Clock
  Data Store Memory : DataStoreMemory  DataStoreName=t3_2
  Data Store Read : DataStoreRead  DataStoreName=t3_2
  Data Store Write : DataStoreWrite  DataStoreName=t3_2
  Element Exponential : Subsystem  mask(Element Exponential){}
      mask help:
      | <p>Возвращает вероятность безотказной работы невосстанавливаемого элемента
      | по экспоненциальному закону распределения.</p>
      | <p>Экспоненциальное (или показательное) распределение — абсолютно непрерывное
      | распределение, моделирующее время между двумя последовательными свершениями
      | одного и того же события.</p>
      | <p>Экспоненциальное распределение используют при оценке надежности сложных
      | технических систем, не подверженных износу и старению и в случаях, когда
      | отказы объектов имеют случайный характер.</p>
      mask Help:
      | <p>Возвращает вероятность безотказной работы невосстанавливаемого элемента по экспоненциальному
      | закону распределения.</p>
      | <p>Экспоненциальное распределение используют при оценке надежности сложных
      | технических систем, не подверженных износу и старению и в случаях, когда
      | отказы объектов имеют случайный характер.</p>
      | <p>Входной параметр λ - интенсивность событий в рассматриваемом потоке.</p>
      | <p>Выходной параметр P(t) - вероятность безотказной работы элемента.</p>
      mask Display:
      | image('images/png/exp.png')
      | port_label('input', 1, 'λ')
      | port_label('output', 1, 'P(t)')
  Element Normal : Subsystem  mask(Element Normal){}
      mask help:
      | <p>Возвращает вероятность безотказной работы невосстанавливаемого
      | элемента по нормальному закону распределения.</p>
      | <p>Нормальное распределение, также называемое распределением Гаусса или
      | Гаусса — Лапласа — распределение вероятностей, которое в одномерном
      | случае задаётся функцией плотности вероятности, совпадающей с функцией
      | Гаусса.</p>
      | <p>Нормальное распределение обычно используют при оценке надежности объектов,
      | основной причиной отказа которых является износ.</p>
      mask Help:
      | <p>Возвращает вероятность безотказной работы невосстанавливаемого
      | элемента по нормальному закону распределения.</p>
      | <p>Нормальное распределение обычно используют при оценке надежности объектов,
      | основной причиной отказа которых является износ.</p>
      | <p>Входные параметры:</p>
      | <p>λ - среднее квадратическое отклонение наработки до отказа,</p>
      | <p>М - математическое ожидание наработки до отказа.</p>
      | <p>Выходной параметр P(t) - вероятность безотказной работы элемента.</p>
      mask Display:
      | image('images/png/normal_nogrid.png')
      | port_label('input', 1, 'λ')
      | port_label('input', 2, 'M')
      | port_label('output', 1, 'P(t)')
  Сircuit Series : Subsystem  mask(Сircuit Series){}
      mask help:
      | <p>Возвращает вероятность безотказной работы двух последовательно соединенных
      | элементов.</p>
      | <p>В системе с последовательной структурой отказ любого компонента приводит
      | к отказу системы в целом.</p>
      mask Help:
      | <p>Возвращает вероятность безотказной работы двух последовательно соединенных
      | элементов.</p>
      | <p>Входные параметры:</p>
      | <p>P1 - вероятность безотказной работы первого элемента,</p>
      | <p>P2 - вероятность безотказной работы второго элемента.</p>
      | <p>Выходной параметр P12 - вероятность безотказной работы двух последовательно
      | соединенных элементов.</p>
      mask Display:
      | image('images/png/series2.png')
      | port_label('input', 1, 'P1')
      | port_label('input', 2, 'P2')
      | port_label('output', 1, 'P12')
  P : Outport
  wires:
  t_start/1 -> Chart/1(t_start)
  Chart/1(tv) -> Data Store Write/1
  Data Store Read/1 -> Element Normal/3(t), Element Exponential/2(t)
  trec/1 -> Chart/4(trec)
  M/1 -> Element Normal/2("M ")
  dP/1 -> Chart/5(dP)
  Pz/1 -> Chart/3(Pz)
  λ1/1 -> Element Exponential/1("lambda ")
  dt/1 -> Chart/2(delta_t)
  Сircuit Series/1(P12) -> Chart/7(P0)
  Clock/1 -> Chart/6(t)
  λ2/1 -> Element Normal/1("lambda ")
  Chart/2(P) -> P/1
  Element Normal/1(P(t)) -> Сircuit Series/2(P2)
  Element Exponential/1(P(t)1) -> Сircuit Series/1(P1)
